simulink library "libturbines"  (R2025b)
settings: Solver=ode45  StartTime=0.0  StopTime=10.0  RelTol=1e-3  EnableMultiTasking=on
undefined symbols (not defined in the file): DiscIntNeverNeededParam, dt, faultOptions, noiseFlag
libraries: simulink x57, $bdroot x3
(part 5 of 5)

== matlab function libturbines/Floating IEA3.4MW faulty/Pitch Actuator/Pitch actuator fault ==
  data: beta input; beta_prev input; PitchActFault input; drift_aux_in input; beta_real output; faultOptions parameter; drift_aux_out output
function [beta_real,drift_aux_out] = fcn(beta,beta_prev,PitchActFault,drift_aux_in,faultOptions)
%%%%%%%%%%%%%%%%%%%%%%%%%%%%%%%%%%%%%%%%%%%%%%%%%%%%%%%%%%%%%%%%%%%%%%%%%
% Pitch actuator fault function
% Inputs:
%   - beta:         Desired pitch angle [deg] from the pitch controller
%   - beta_meas:    Actual pitch angle (measured) [deg]
%   - fault_type:   Desired fault type:
%                     0 - no fault
%                     1 - stuck at a fixed value
%                     2 - constant offset fault
%                     3 - drifting actuator
%                     4 - constant gain fault
%                     5 - change of actuator dynamics (in a different function)
% Outputs:
%   - beta_real:    Real pitch angle [deg] after the effect of the fault
%
%
% Author: Yerai Peña-Sanchez
%%%%%%%%%%%%%%%%%%%%%%%%%%%%%%%%%%%%%%%%%%%%%%%%%%%%%%%%%%%%%%%%%%%%%%%%

y_t = beta;  % Without any fault
switch floor(PitchActFault)
    case 1  % Stuck at a fixed value
        y_t(3) = beta_prev(3);
    case 2  % Constant offset value
        y_t(3) = y_t(3)-faultOptions.PitchActOffset;
    case 3  % Drifting value
        drift_aux_in = drift_aux_in + 1;
        y_t(3) = y_t(3) + drift_aux_in*faultOptions.PitchActDriftSlope;
    case 4  % Constant gain
        y_t(3) = y_t(3)*faultOptions.PitchActGain;
end

if floor(PitchActFault) ~= 3
    drift_aux_out = 0;
else
    drift_aux_out = drift_aux_in;
end

% beta_real = [y_t; beta; beta];
beta_real = y_t;

== matlab function libturbines/Floating IEA3.4MW faulty/Sensors sampling/Generator power sensor fault ==
  settings: updateMethod=DISCRETE
  data: p_gen_real input; p_gen_prev input; GenPSenFault input; drift_aux_in input; p_gen_meas output; faultOptions parameter; drift_aux_out output
function [p_gen_meas,drift_aux_out] = fcn(p_gen_real,p_gen_prev,GenPSenFault,drift_aux_in,faultOptions)
%%%%%%%%%%%%%%%%%%%%%%%%%%%%%%%%%%%%%%%%%%%%%%%%%%%%%%%%%%%%%%%%%%%%%%%%%
% Generator power sensor fault function
% Inputs:
%   - p_gen_real:   Real generator power [W]
%   - p_gen_prev:   Previous generator power (measured) [W]
%   - fault_type:   Desired fault type:
%                     0 - no fault
%                     1 - stuck at a fixed value
%                     2 - constant offset fault
%                     3 - drifting fault
%                     4 - constant gain fault
%                     5 - loss of precision
% Outputs:
%   - p_gen_meas:   Measured generator power [W] after the effect of the fault
%
%
% Author: Yerai Peña-Sanchez
%%%%%%%%%%%%%%%%%%%%%%%%%%%%%%%%%%%%%%%%%%%%%%%%%%%%%%%%%%%%%%%%%%%%%%%%

y_t = p_gen_real;  % Without any fault
switch floor(GenPSenFault)
    case 1  % Stuck at a fixed value
        y_t = p_gen_prev;
    case 2  % Constant offset value
        y_t = p_gen_real-faultOptions.GenPSenOffset;
    case 3  % Drifting value
        drift_aux_in = drift_aux_in + 1;
        y_t = p_gen_real + drift_aux_in*faultOptions.GenPSenDriftSlope;
    case 4  % Constant gain value
        y_t = p_gen_real*faultOptions.GenPSenGain;
    case 5  % Loss of precision of the sensor
        y_t = p_gen_real+p_gen_real*(2*rand-1)*faultOptions.GenPSenPrecision;
end

if floor(GenPSenFault) ~= 3
    drift_aux_out = 0;
else
    drift_aux_out = drift_aux_in;
end
p_gen_meas = y_t;

== matlab function libturbines/Floating IEA3.4MW faulty/Sensors sampling/Generator speed sensor fault ==
  settings: updateMethod=DISCRETE
  data: w_gen_real input; w_gen_prev input; GenSenFault input; drift_aux_in input; w_gen_meas output; faultOptions parameter; drift_aux_out output
function [w_gen_meas,drift_aux_out] = fcn(w_gen_real,w_gen_prev,GenSenFault,drift_aux_in,faultOptions)
%%%%%%%%%%%%%%%%%%%%%%%%%%%%%%%%%%%%%%%%%%%%%%%%%%%%%%%%%%%%%%%%%%%%%%%%%
% Generator speed sensor fault function
% Inputs:
%   - w_gen_real:   Real generator speed [rad/s]
%   - w_gen_prev:   Previous generator speed (measured) [rad/s]
%   - fault_type:   Desired fault type:
%                     0 - no fault
%                     1 - stuck at a fixed value
%                     2 - constant offset fault
%                     3 - drifting fault
%                     4 - constant gain fault
%                     5 - loss of precision
% Outputs:
%   - w_gen_meas:   Measured generator speed [rad/s] after the effect of the fault
%
%
% Author: Yerai Peña-Sanchez
%%%%%%%%%%%%%%%%%%%%%%%%%%%%%%%%%%%%%%%%%%%%%%%%%%%%%%%%%%%%%%%%%%%%%%%%

y_t = w_gen_real;  % Without any fault
switch floor(GenSenFault)
    case 1  % Stuck at a fixed value
        y_t = w_gen_prev;
    case 2  % Constant offset value
        y_t = w_gen_real-faultOptions.GenSenOffset;
    case 3  % Drifting value
        drift_aux_in = drift_aux_in + 1;
        y_t = w_gen_real + drift_aux_in*faultOptions.GenSenDriftSlope;
    case 4  % Constant gain value
        y_t = w_gen_real*faultOptions.GenSenGain;
    case 5  % Loss of precision of the sensor
        y_t = w_gen_real+w_gen_real*(2*rand-1)*faultOptions.GenSenPrecision;
end

if floor(GenSenFault) ~= 3
    drift_aux_out = 0;
else
    drift_aux_out = drift_aux_in;
end
w_gen_meas = y_t;

== matlab function libturbines/Floating IEA3.4MW faulty/Sensors sampling/Pitch sensor fault ==
  settings: updateMethod=DISCRETE
  data: beta_real input; beta_prev input; PitchSenFault input; drift_aux_in input; beta_meas output; faultOptions parameter; drift_aux_out output
function [beta_meas,drift_aux_out] = fcn(beta_real,beta_prev,PitchSenFault,drift_aux_in,faultOptions)
%%%%%%%%%%%%%%%%%%%%%%%%%%%%%%%%%%%%%%%%%%%%%%%%%%%%%%%%%%%%%%%%%%%%%%%%%
% Pitch sensor fault function
% Inputs:
%   - beta_real:    Real pitch angle [deg] of the actuator
%   - beta_prev:    Previous pitch angle (measured) [deg]
%   - fault_type:   Desired fault type:
%                     0 - no fault
%                     1 - stuck at a fixed value
%                     2 - constant offset fault
%                     3 - drifting fault
%                     4 - constant gain fault
%                     5 - loss of precision
% Outputs:
%   - beta_meas:    Measured pitch angle [deg] after the effect of the fault
%
%
% Author: Yerai Peña-Sanchez
%%%%%%%%%%%%%%%%%%%%%%%%%%%%%%%%%%%%%%%%%%%%%%%%%%%%%%%%%%%%%%%%%%%%%%%%

y_t = beta_real;  % Without any fault
switch floor(PitchSenFault)
    case 1  % Stuck at a fixed value
        y_t(3) = beta_prev(3);
    case 2  % Constant offset value
        y_t(3) = beta_real(3)-faultOptions.PitchSenOffset;
    case 3  % Drifting value
        drift_aux_in = drift_aux_in + 1;
        y_t(3) = beta_real(3) + drift_aux_in*faultOptions.PitchSenDriftSlope;
    case 4  % Constant gain value
        y_t(3) = beta_real(3)*faultOptions.PitchSenGain;
    case 5  % Loss of precision of the sensor
        y_t(3) = beta_real(3)+beta_real(3)*(2*rand-1)*faultOptions.PitchSenPrecision;
end

if floor(PitchSenFault) ~= 3
    drift_aux_out = 0;
else
    drift_aux_out = drift_aux_in;
end
% beta_meas = [y_t; beta_real; beta_real];
beta_meas = y_t;

== matlab function libturbines/Floating IEA3.4MW faulty/Sensors sampling/Rotor speed sensor fault ==
  settings: updateMethod=DISCRETE
  data: w_rot_real input; w_rot_prev input; RotSenFault input; drift_aux_in input; w_rot_meas output; faultOptions parameter; drift_aux_out output
function [w_rot_meas,drift_aux_out] = fcn(w_rot_real,w_rot_prev,RotSenFault,drift_aux_in,faultOptions)
%%%%%%%%%%%%%%%%%%%%%%%%%%%%%%%%%%%%%%%%%%%%%%%%%%%%%%%%%%%%%%%%%%%%%%%%%
% Rotor speed sensor fault function
% Inputs:
%   - w_gen_real:   Real rotor speed [rad/s]
%   - w_gen_prev:   Previous generator speed (measured) [rad/s]
%   - fault_type:   Desired fault type:
%                     0 - no fault
%                     1 - stuck at a fixed value
%                     2 - constant offset fault
%                     3 - drifting fault
%                     4 - constant gain fault
%                     5 - loss of precision
% Outputs:
%   - w_rot_meas:   Measured rotor speed [rad/s] after the effect of the fault
%
%
% Author: Yerai Peña-Sanchez
%%%%%%%%%%%%%%%%%%%%%%%%%%%%%%%%%%%%%%%%%%%%%%%%%%%%%%%%%%%%%%%%%%%%%%%%

y_t = w_rot_real;  % Without any fault
switch floor(RotSenFault)
    case 1  % Stuck at a fixed value
        y_t = w_rot_prev;
    case 2  % Constant offset value
        y_t = w_rot_real-faultOptions.RotSenOffset;
    case 3  % Drifting value
        drift_aux_in = drift_aux_in + 1;
        y_t = w_rot_real + drift_aux_in*faultOptions.RotSenDriftSlope;
    case 4  % Constant gain value
        y_t = w_rot_real*faultOptions.RotSenGain;
    case 5  % Loss of precision of the sensor
        y_t = w_rot_real+w_rot_real*(2*rand-1)*faultOptions.RotSenPrecision;
end

if floor(RotSenFault) ~= 3
    drift_aux_out = 0;
else
    drift_aux_out = drift_aux_in;
end
w_rot_meas = y_t;

== matlab function libturbines/Floating IEA15MW faulty/Generator simple/Generator fault ==
  data: GenActFault input; torque input; torque_prev input; drift_aux_in input; torque_real output; faultOptions parameter; drift_aux_out output
function [torque_real,drift_aux_out] = fcn(GenActFault,torque,torque_prev,drift_aux_in,faultOptions)
%%%%%%%%%%%%%%%%%%%%%%%%%%%%%%%%%%%%%%%%%%%%%%%%%%%%%%%%%%%%%%%%%%%%%%%%%
% Generator fault function
% Inputs:
%   - torque:       Reference torque value [Nm] from the controller
%   - fault_type:   Desired fault type:
%                     0 - no fault
%                     1 - stuck at a fixed value
%                     2 - constant offset fault
%                     3 - loss of efectiveness (in a different function)
% Outputs:
%   - torque_real:  Real torque value [Nm] after the effect of the fault
%
%
% Author: Yerai Peña-Sanchez
%%%%%%%%%%%%%%%%%%%%%%%%%%%%%%%%%%%%%%%%%%%%%%%%%%%%%%%%%%%%%%%%%%%%%%%%

y_t = torque;  % Without any fault
switch floor(GenActFault)
    case 1  % Stuck generator
        y_t = torque_prev;
    case 2  % Constant offset value
        y_t = y_t-faultOptions.GenActOffset;
    case 3  % Drifting value
        drift_aux_in = drift_aux_in + 1;
        y_t = y_t + drift_aux_in*faultOptions.GenActDriftSlope;
    case 4  % Constant gain value
        y_t = y_t*faultOptions.GenActGain;
end

if floor(GenActFault) ~= 3
    drift_aux_out = 0;
else
    drift_aux_out = drift_aux_in;
end

torque_real = y_t;

== matlab function libturbines/Floating NREL5MW faulty/Generator simple/Generator fault ==
  data: GenActFault input; torque input; torque_prev input; drift_aux_in input; torque_real output; faultOptions parameter; drift_aux_out output
function [torque_real,drift_aux_out] = fcn(GenActFault,torque,torque_prev,drift_aux_in,faultOptions)
%%%%%%%%%%%%%%%%%%%%%%%%%%%%%%%%%%%%%%%%%%%%%%%%%%%%%%%%%%%%%%%%%%%%%%%%%
% Generator fault function
% Inputs:
%   - torque:       Reference torque value [Nm] from the controller
%   - fault_type:   Desired fault type:
%                     0 - no fault
%                     1 - stuck at a fixed value
%                     2 - constant offset fault
%                     3 - loss of efectiveness (in a different function)
% Outputs:
%   - torque_real:  Real torque value [Nm] after the effect of the fault
%
%
% Author: Yerai Peña-Sanchez
%%%%%%%%%%%%%%%%%%%%%%%%%%%%%%%%%%%%%%%%%%%%%%%%%%%%%%%%%%%%%%%%%%%%%%%%

y_t = torque;  % Without any fault
switch floor(GenActFault)
    case 1  % Stuck generator
        y_t = torque_prev;
    case 2  % Constant offset value
        y_t = y_t-faultOptions.GenActOffset;
    case 3  % Drifting value
        drift_aux_in = drift_aux_in + 1;
        y_t = y_t + drift_aux_in*faultOptions.GenActDriftSlope;
    case 4  % Constant gain value
        y_t = y_t*faultOptions.GenActGain;
end

if floor(GenActFault) ~= 3
    drift_aux_out = 0;
else
    drift_aux_out = drift_aux_in;
end

torque_real = y_t;

== matlab function libturbines/Floating NREL5MW faulty/Generator simple/Generator fault type 3 ==
  data: GenActFault input; out output; faultOptions parameter
function out = fcn(GenActFault,faultOptions)
%%%%%%%%%%%%%%%%%%%%%%%%%%%%%%%%%%%%%%%%%%%%%%%%%%%%%%%%%%%%%%%%%%%%%%%%%
% Generator loss of effectiveness fault type signal generator
% Inputs:
%   - fault_type:   Desired fault type:
%                     0 - no fault
%                     1 - stuck at a fixed value (in a different function)
%                     2 - constant offset fault (in a different function)
%                     3 - loss of efectiveness
% Outputs:
%   - out:          Signal for the loss of effectiveness fault and the faulty signal
%
%
% Author: Yerai Peña-Sanchez
%%%%%%%%%%%%%%%%%%%%%%%%%%%%%%%%%%%%%%%%%%%%%%%%%%%%%%%%%%%%%%%%%%%%%%%%

out = [GenActFault ; 1];              % Without any fault
if GenActFault == 3                   % Loss of effectiveness fault
    out(2) = faultOptions.GenActEffectiveness;
end

== matlab function libturbines/Floating IEA15MW faulty/Generator simple/Generator fault type 3 ==
  data: GenActFault input; out output; faultOptions parameter
function out = fcn(GenActFault,faultOptions)
%%%%%%%%%%%%%%%%%%%%%%%%%%%%%%%%%%%%%%%%%%%%%%%%%%%%%%%%%%%%%%%%%%%%%%%%%
% Generator loss of effectiveness fault type signal generator
% Inputs:
%   - fault_type:   Desired fault type:
%                     0 - no fault
%                     1 - stuck at a fixed value (in a different function)
%                     2 - constant offset fault (in a different function)
%                     3 - loss of efectiveness
% Outputs:
%   - out:          Signal for the loss of effectiveness fault and the faulty signal
%
%
% Author: Yerai Peña-Sanchez
%%%%%%%%%%%%%%%%%%%%%%%%%%%%%%%%%%%%%%%%%%%%%%%%%%%%%%%%%%%%%%%%%%%%%%%%

out = [GenActFault ; 1];              % Without any fault
if GenActFault == 3                   % Loss of effectiveness fault
    out(2) = faultOptions.GenActEffectiveness;
end

== matlab function libturbines/Floating NREL5MW faulty/Pitch Actuator/Pitch actuator fault ==
  data: beta input; beta_prev input; PitchActFault input; drift_aux_in input; beta_real output; faultOptions parameter; drift_aux_out output
function [beta_real,drift_aux_out] = fcn(beta,beta_prev,PitchActFault,drift_aux_in,faultOptions)
%%%%%%%%%%%%%%%%%%%%%%%%%%%%%%%%%%%%%%%%%%%%%%%%%%%%%%%%%%%%%%%%%%%%%%%%%
% Pitch actuator fault function
% Inputs:
%   - beta:         Desired pitch angle [deg] from the pitch controller
%   - beta_meas:    Actual pitch angle (measured) [deg]
%   - fault_type:   Desired fault type:
%                     0 - no fault
%                     1 - stuck at a fixed value
%                     2 - constant offset fault
%                     3 - drifting actuator
%                     4 - constant gain fault
%                     5 - change of actuator dynamics (in a different function)
% Outputs:
%   - beta_real:    Real pitch angle [deg] after the effect of the fault
%
%
% Author: Yerai Peña-Sanchez
%%%%%%%%%%%%%%%%%%%%%%%%%%%%%%%%%%%%%%%%%%%%%%%%%%%%%%%%%%%%%%%%%%%%%%%%

y_t = beta;  % Without any fault
switch floor(PitchActFault)
    case 1  % Stuck at a fixed value
        y_t(3) = beta_prev(3);
    case 2  % Constant offset value
        y_t(3) = y_t(3)-faultOptions.PitchActOffset;
    case 3  % Drifting value
        drift_aux_in = drift_aux_in + 1;
        y_t(3) = y_t(3) + drift_aux_in*faultOptions.PitchActDriftSlope;
    case 4  % Constant gain
        y_t(3) = y_t(3)*faultOptions.PitchActGain;
end

if floor(PitchActFault) ~= 3
    drift_aux_out = 0;
else
    drift_aux_out = drift_aux_in;
end

% beta_real = [y_t; beta; beta];
beta_real = y_t;

== matlab function libturbines/Floating NREL5MW faulty/Sensors sampling/Pitch sensor fault ==
  settings: updateMethod=DISCRETE
  data: beta_real input; beta_prev input; PitchSenFault input; drift_aux_in input; beta_meas output; faultOptions parameter; drift_aux_out output
function [beta_meas,drift_aux_out] = fcn(beta_real,beta_prev,PitchSenFault,drift_aux_in,faultOptions)
%%%%%%%%%%%%%%%%%%%%%%%%%%%%%%%%%%%%%%%%%%%%%%%%%%%%%%%%%%%%%%%%%%%%%%%%%
% Pitch sensor fault function
% Inputs:
%   - beta_real:    Real pitch angle [deg] of the actuator
%   - beta_prev:    Previous pitch angle (measured) [deg]
%   - fault_type:   Desired fault type:
%                     0 - no fault
%                     1 - stuck at a fixed value
%                     2 - constant offset fault
%                     3 - drifting fault
%                     4 - constant gain fault
%                     5 - loss of precision
% Outputs:
%   - beta_meas:    Measured pitch angle [deg] after the effect of the fault
%
%
% Author: Yerai Peña-Sanchez
%%%%%%%%%%%%%%%%%%%%%%%%%%%%%%%%%%%%%%%%%%%%%%%%%%%%%%%%%%%%%%%%%%%%%%%%

y_t = beta_real;  % Without any fault
switch floor(PitchSenFault)
    case 1  % Stuck at a fixed value
        y_t(3) = beta_prev(3);
    case 2  % Constant offset value
        y_t(3) = beta_real(3)-faultOptions.PitchSenOffset;
    case 3  % Drifting value
        drift_aux_in = drift_aux_in + 1;
        y_t(3) = beta_real(3) + drift_aux_in*faultOptions.PitchSenDriftSlope;
    case 4  % Constant gain value
        y_t(3) = beta_real(3)*faultOptions.PitchSenGain;
    case 5  % Loss of precision of the sensor
        y_t(3) = beta_real(3)+beta_real(3)*(2*rand-1)*faultOptions.PitchSenPrecision;
end

if floor(PitchSenFault) ~= 3
    drift_aux_out = 0;
else
    drift_aux_out = drift_aux_in;
end
% beta_meas = [y_t; beta_real; beta_real];
beta_meas = y_t;

== matlab function libturbines/Floating IEA15MW faulty/Pitch Actuator/Pitch actuator fault ==
  data: beta input; beta_prev input; PitchActFault input; drift_aux_in input; beta_real output; faultOptions parameter; drift_aux_out output
function [beta_real,drift_aux_out] = fcn(beta,beta_prev,PitchActFault,drift_aux_in,faultOptions)
%%%%%%%%%%%%%%%%%%%%%%%%%%%%%%%%%%%%%%%%%%%%%%%%%%%%%%%%%%%%%%%%%%%%%%%%%
% Pitch actuator fault function
% Inputs:
%   - beta:         Desired pitch angle [deg] from the pitch controller
%   - beta_meas:    Actual pitch angle (measured) [deg]
%   - fault_type:   Desired fault type:
%                     0 - no fault
%                     1 - stuck at a fixed value
%                     2 - constant offset fault
%                     3 - drifting actuator
%                     4 - constant gain fault
%                     5 - change of actuator dynamics (in a different function)
% Outputs:
%   - beta_real:    Real pitch angle [deg] after the effect of the fault
%
%
% Author: Yerai Peña-Sanchez
%%%%%%%%%%%%%%%%%%%%%%%%%%%%%%%%%%%%%%%%%%%%%%%%%%%%%%%%%%%%%%%%%%%%%%%%

y_t = beta;  % Without any fault
switch floor(PitchActFault)
    case 1  % Stuck at a fixed value
        y_t(3) = beta_prev(3);
    case 2  % Constant offset value
        y_t(3) = y_t(3)-faultOptions.PitchActOffset;
    case 3  % Drifting value
        drift_aux_in = drift_aux_in + 1;
        y_t(3) = y_t(3) + drift_aux_in*faultOptions.PitchActDriftSlope;
    case 4  % Constant gain
        y_t(3) = y_t(3)*faultOptions.PitchActGain;
end

if floor(PitchActFault) ~= 3
    drift_aux_out = 0;
else
    drift_aux_out = drift_aux_in;
end

% beta_real = [y_t; beta; beta];
beta_real = y_t;
